simulink model "PV_Boost_VSI_Ilhamento_SMS_2023b"  (R2024b)
settings: Solver=ode4  StartTime=0  StopTime=5  FixedStep=1e-6  MaxStep=1e-6  RelTol=0.1e-3
undefined symbols (not defined in the file): Cl, Ll, Rl
libraries: spsSeriesRLCBranchLib x7, spsIGBTDiodeLib x5, spsGroundLib x4, spsVoltageMeasurementLib x4, slpidlib x3, simulink x3, spsBreakerLib x2, spsCurrentMeasurementLib x2, spsDiodeLib x2, spsMeanLib x2, spsACVoltageSourceLib x1, spsParallelRLCBranchLib x1
settings Model: SimulationMode=accelerator  Creator=rodrigo  LastModifiedBy=aleks
settings SolverCC: MaxConsecutiveZCs=10000  ShapePreserveControl=EnableAll  ZeroCrossControl=EnableAll
settings DataIOCC: SaveFormat=Array  SignalLoggingSaveFormat=ModelDataLogs  SaveOutput=off  SaveTime=off  ReturnWorkspaceOutputs=off
settings OptimizationCC: BooleanDataType=off  ExpressionDepthLimit=2147483647  InitFltsAndDblsToZero=on  EfficientMapNaN2IntZero=off  LifeSpan=inf  AccelVerboseBuild=on
settings DebuggingCC: SaveWithParameterizedLinksMsg=none  UnderspecifiedInitializationDetection=Classic  MergeDetectMultiDrivingBlocksExec=none  SignalResolutionControl=TryResolveAllWithWarning  MultiTaskDSMMsg=warning  MultiTaskCondExecSysMsg=none  FcnCallInpInsideContextMsg=warning  UnconnectedInputMsg=warning  UnconnectedOutputMsg=warning  UnconnectedLineMsg=warning  StateNameClashWarn=warning  StrictBusMsg=WarnOnBusTreatedAsVector  SFUnexpectedBacktrackingDiag=warning  SFNoUnconditionalDefaultTransitionDiag=warning  SFExecutionAtInitializationDiag=none  ArithmeticOperatorsInVariantConditions=warning
settings HardwareCC: ProdBitPerPointer=32  ProdBitPerSizeT=32  ProdBitPerPtrDiffT=32  ProdLargestAtomicFloat=None  ProdIntDivRoundTo=Undefined  ProdEndianess=Unspecified  ProdWordSize=32  ProdHWDeviceType=32-bit Generic  TargetBitPerPointer=64  TargetBitPerSizeT=64  TargetBitPerPtrDiffT=64  TargetLongLongMode=on  TargetIntDivRoundTo=Zero  TargetEndianess=LittleEndian  TargetWordSize=64  TargetHWDeviceType=MATLAB Host  ProdEqTarget=off
settings ModelReferenceCC: PropagateSignalLabelsOutOfModel=off
settings SFSimCC: SimUseLocalCustomCode=off  SimParseCustomCode=off  CustomCodeUndefinedFunction=UseInterfaceOnly
settings RTWCC: RTWUseLocalCustomCode=off  GPUComputeCapability=3.5
settings CodeAppCC: MaxIdLength=128  StateflowObjectComments=on
settings GRTTargetCC: TargetLangStandard=C89/C90 (ANSI)  CombineOutputUpdateFcns=off  GRTInterface=on
settings ConfigComp: CovMetricSettings=dw  CovSaveCumulativeToWorkspaceVar=on  CovSaveSingleToWorkspaceVar=on  CovExternalEMLEnable=off  DVMaxTestCaseSteps=500  DVTestSuiteOptimization=CombinedObjectives (Nonlinear Extended)  DVDefectChecker=off  DVDetectActiveLogic=on  DVHarnessSource=Signal Editor
settings SimscapeCC: SimscapeNormalizeSystem=off

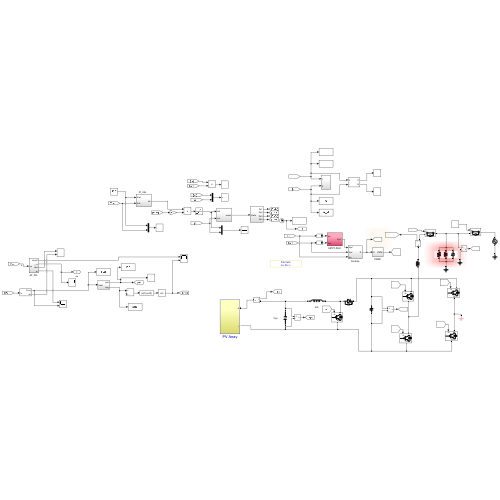
[thumbnail: Simulink's stored preview of the top-level diagram]
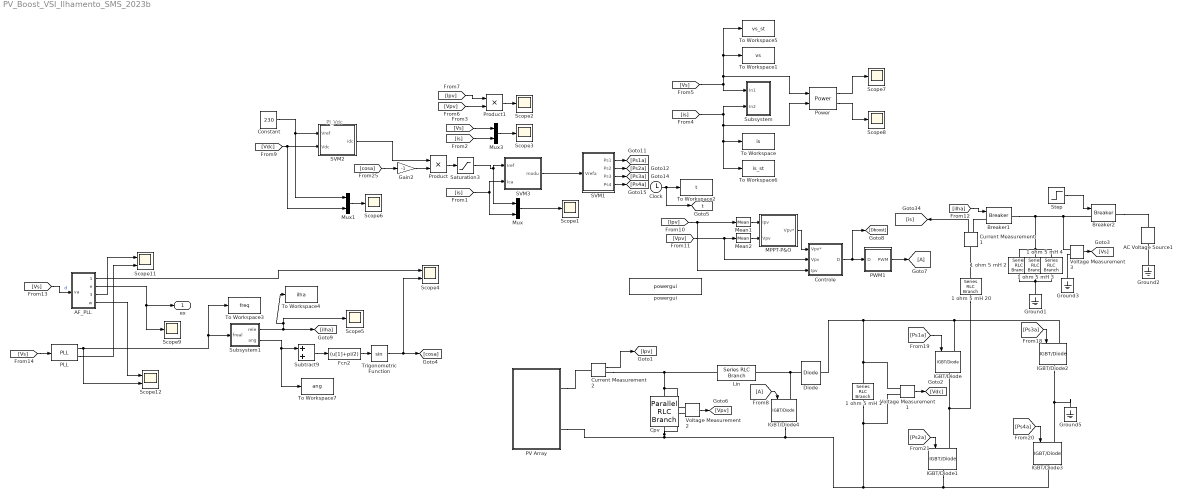
== system PV_Boost_VSI_Ilhamento_SMS_2023b ==
  note: PI_Vdc
  1 ohm 5 mH 1 : spsSeriesRLCBranchLib/Series RLC Branch  LConnTagsString=__new0  RConnTagsString=__new0  BranchType=C  Resistance=100  Inductance=0.547e-3  SetiL0=off  InitialCurrent=10  Capacitance=0.002115  Setx0=on  InitialVoltage=230  Measurements=None
  1 ohm 5 mH 2 : spsSeriesRLCBranchLib/Series RLC Branch  LConnTagsString=__new0  RConnTagsString=__new0  BranchType=R  Resistance=Rl  Inductance=5e-03  SetiL0=off  InitialCurrent=0  Capacitance=0.001  Setx0=off  InitialVoltage=0  Measurements=None
  1 ohm 5 mH 20 : spsSeriesRLCBranchLib/Series RLC Branch  LConnTagsString=__new0  RConnTagsString=__new0  BranchType=L  Resistance=100  Inductance=1.5e-3  SetiL0=off  InitialCurrent=10  Capacitance=60u  Setx0=off  InitialVoltage=0  Measurements=None
  1 ohm 5 mH 3 : spsSeriesRLCBranchLib/Series RLC Branch  LConnTagsString=__new0  RConnTagsString=__new0  BranchType=L  Resistance=100  Inductance=Ll  SetiL0=off  InitialCurrent=10  Capacitance=60u  Setx0=off  InitialVoltage=0  Measurements=None
  1 ohm 5 mH 4 : spsSeriesRLCBranchLib/Series RLC Branch  LConnTagsString=__new0  RConnTagsString=__new0  BranchType=C  Resistance=100  Inductance=0.547e-3  SetiL0=off  InitialCurrent=10  Capacitance=Cl  Setx0=off  InitialVoltage=230  Measurements=None
  AC Voltage Source1 : spsACVoltageSourceLib/AC Voltage Source  Amplitude=127*sqrt(2)  Phase=0  Frequency=60  SampleTime=0  Measurements=None  BusType=swing  Pref=10e3  Qref=0  Qmin=-inf  Qmax=+inf
  AF_PLL : Subsystem
  Breaker1 : spsBreakerLib/Breaker  InitialState=1  SwitchingTimes="[1/60  5/60]"  External=on  BreakerResistance=0.0001  SnubberResistance=1e6  SnubberCapacitance=inf  Measurements=None  MoreParameters=on  NoBreakLoop=off
  Breaker2 : spsBreakerLib/Breaker  InitialState=1  SwitchingTimes="[1/60  5/60]"  External=on  BreakerResistance=0.0001  SnubberResistance=1e6  SnubberCapacitance=inf  Measurements=None  MoreParameters=on  NoBreakLoop=off
  Clock : Clock
  Constant : Constant  Value=230  SampleTime=-1
  Controle : Subsystem
  Cpv : spsParallelRLCBranchLib/Parallel RLC Branch  LConnTagsString=a  RConnTagsString=__new0  BranchType=C  Resistance=1  Inductance=1e-3  SetiL0=off  InitialCurrent=0  Capacitance=100e-6  Setx0=off  InitialVoltage=0  Measurements=Branch voltage
  Current Measurement1 : spsCurrentMeasurementLib/Current Measurement  PhasorSimulation=off  OutputType=Complex  PSBequivalent=0
  Current Measurement2 : spsCurrentMeasurementLib/Current Measurement  PhasorSimulation=off  OutputType=Complex  PSBequivalent=0
  Diode : spsDiodeLib/Diode  Ron=0.001  Lon=0  Vf=0.0  IC=0  UseSnubber=off  Rs=500  Cs=250e-9  Measurements=off
  Fcn2 : Fcn  Expr=(u[1]+pi/2)
  From8 : From
  Gain2 : Gain  Gain=-1
  Goto7 : Goto
  Ground{1..3,5} (4 alike) : spsGroundLib/Ground  LConnTagsString=a
  IGBT/Diode{,1..4} (5 alike) : spsIGBTDiodeLib/IGBT//Diode  Ron=1e-3  Rs=1e5  Cs=inf  Measurements=off
  Lin : spsSeriesRLCBranchLib/Series RLC Branch  LConnTagsString=__new0  RConnTagsString=__new0  BranchType=L  Resistance=0.01  Inductance=2.5e-3  SetiL0=off  InitialCurrent=0  Capacitance=1e-6  Setx0=off  InitialVoltage=0  Measurements=Branch current
  MPPT-P&O : Subsystem
  Mean1 : spsMeanLib/Mean  Freq=200  Vinit=0  Ts=0
  Mean2 : spsMeanLib/Mean  Freq=200  Vinit=0  Ts=0
  Mux : Mux  Inputs=2
  Mux1 : Mux  Inputs=2
  Mux3 : Mux  Inputs=2
  PLL : spsPLLLib/PLL  Fmin=45  Par_Init=[0, 60]  ParK=[180, 3200, 1]  TcD=1e-4  MaxRateChangeFreq=12  FilterCutOffFreq=25  Ts=0  AGC=on
      settings: LibrarySourceBlock=sps_lib/Control/PLL
  PV Array : Subsystem
  PWM1 : Subsystem
  Power : spsPowerLib/Power  Freq=60  Vinit=[1, 0]  Iinit=[1, 0]  Ts=0
  Product : Product  RndMeth=Zero
  Product1 : Product  RndMeth=Zero
  SVM1 : Subsystem
  SVM2 : Subsystem
  SVM3 : Subsystem
  Saturation3 : Saturate  UpperLimit=1000  LowerLimit=-100  LinearizeAsGain=off
  Scope{1..3,5..9} (8 alike) : Scope
  Scope11 : Scope  NumInputPorts=2
  Scope12 : Scope  NumInputPorts=2
  Scope4 : Scope  NumInputPorts=2
  Step : Step  Time=3  Before=1  After=0  SampleTime=0
  Subsystem : Subsystem
  Subsystem1 : Subsystem
  Subtract9 : Sum
  To Workspace : ToWorkspace  VariableName=is  SampleTime=-1
      settings: Decimation=100
  To Workspace1 : ToWorkspace  VariableName=vs  SampleTime=-1
      settings: Decimation=100
  To Workspace2 : ToWorkspace  VariableName=t  SampleTime=1e-6
      settings: Decimation=100
  To Workspace3 : ToWorkspace  VariableName=freq  SampleTime=-1
      settings: Decimation=100
  To Workspace4 : ToWorkspace  VariableName=ilha  SampleTime=-1
      settings: Decimation=100
  To Workspace5 : ToWorkspace  VariableName=vs_st  SaveFormat=Structure With Time  SampleTime=-1
      settings: Decimation=100
  To Workspace6 : ToWorkspace  VariableName=is_st  SaveFormat=Structure With Time  SampleTime=-1
      settings: Decimation=100
  To Workspace7 : ToWorkspace  VariableName=ang  SampleTime=-1
      settings: Decimation=100
  Trigonometric Function : Trigonometry
  Voltage Measurement1 : spsVoltageMeasurementLib/Voltage Measurement  PhasorSimulation=off  OutputType=Complex  PSBequivalent=0
  Voltage Measurement2 : spsVoltageMeasurementLib/Voltage Measurement  PhasorSimulation=off  OutputType=Complex  PSBequivalent=0
  Voltage Measurement3 : spsVoltageMeasurementLib/Voltage Measurement  PhasorSimulation=off  OutputType=Complex  PSBequivalent=0
  powergui : spspowerguiLib/powergui  Priority=1  SimulationMode=Discrete  SampleTime=1e-6  frequency=60  Iterations=50  frequencyindice=0  Pbase=100e6  ErrMax=1e-4  UnitsV=kV  UnitsW=MW  buscounter=0  FunctionMessages=off  echomessages=off  EnableUseOfTLC=off  CurrentSourceSwitches=off  DisableSnubberDevices=off  DisableRonSwitches=off  DisableVfSwitches=off  DisplayEquations=off  AutomaticDiscreteSolvers=off  SolverType=Tustin  Interpol=off  ExternalGateDelay=off  methode=off  Ts=0  x0status=blocks  SPID=on  SwTol=0  HookPort=off  NonlinearTolerance=1e-4  nMaxIteration=100  ContinueOnMaxIteration=off  RestoreLinks=warning  ResistiveCurrentMeasurement=off  Frange=[0:2:500]  Ylog=off  Xlog=on  ShowGrid=off  save=off  variable=ZData  structure=fft  ZoomFFT=on  StartTime=1  cycles=5  DisplayStyle=2  fundamental=60  FreqAxis=on  MaxFrequency=51*60  frequencyindicesteady=1  RmsSteady=1  display=off
  ex : Outport
  tag scope: t=global
  wires:
  [Ps3a] -> IGBT/Diode2/1
  [Ps1a] -> IGBT/Diode/1
  [Ps4a] -> IGBT/Diode3/1
  [Ps2a] -> IGBT/Diode1/1
  SVM1/1(Ps1) -> [Ps1a]
  SVM1/2(Ps2) -> [Ps2a]
  SVM1/3(Ps3) -> [Ps3a]
  SVM1/4(Ps4) -> [Ps4a]
  Voltage Measurement1/1 -> [Vdc]
  [Vdc] -> Mux1/2, SVM2/2(Vdc)
  Saturation3/1 -> SVM3/1(Iref), Mux/1
  Mux/1 -> Scope1/1
  [is] -> Mux/2, SVM3/2(Ica)
  Mux1/1 -> Scope6/1
  Constant/1 -> Mux1/1, SVM2/1(Vref)
  Current Measurement1/1 -> [is]
  Mux3/1 -> Scope3/1
  [is] -> Mux3/2
  Current Measurement2/1 -> [Ipv]
  [Vs] -> Mux3/1
  Product1/1 -> Scope2/1
  [Vpv] -> Product1/2
  [Ipv] -> Product1/1
  From8/1 -> IGBT/Diode4/1
  Voltage Measurement2/1 -> [Vpv]
  Product/1 -> Saturation3/1
  SVM2/1(idc) -> Product/1
  [Vpv] -> Controle/2(Vpv), Mean2/1
  [Ipv] -> Controle/3(Ipv), Mean1/1
  Controle/1(D) -> [Dboost], PWM1/1(D)
  MPPT-P&O/1(Vpv*) -> Controle/1(Vpv*)
  Mean2/1 -> MPPT-P&O/2(Vpv)
  Mean1/1 -> MPPT-P&O/1(Ipv)
  PWM1/1(PWM) -> Goto7/1
  Step/1 -> Breaker2/1
  [Vs] -> To Workspace5/1, To Workspace1/1, Power/1, Subsystem/1(In1)
  [is] -> Subsystem/2(In2), Power/2, To Workspace/1, To Workspace6/1
  Clock/1 -> [t], To Workspace2/1
  [Vs] -> PLL/1
  Gain2/1 -> Product/2
  SVM3/1(modu) -> SVM1/1(Vrefa)
  Trigonometric Function/1 -> [cosa], Scope4/2
  [cosa] -> Gain2/1
  Subsystem1/1(rele) -> To Workspace4/1, Scope5/1, [ilha]
  Power/1 -> Scope7/1
  Power/2 -> Scope8/1
  Subsystem1/2(ang) -> Subtract9/1, To Workspace7/1
  [Vs] -> AF_PLL/1(va)  "d"
  AF_PLL/1(cosa2) -> Scope4/1
  AF_PLL/2(e) -> Scope9/1, ex/1
  Voltage Measurement3/1 -> [Vs]
  [ilha] -> Breaker1/1
  PLL/2 -> Scope11/2
  AF_PLL/4(w) -> Scope12/1
  Subtract9/1 -> Fcn2/1
  Fcn2/1 -> Trigonometric Function/1
  PLL/1 -> To Workspace3/1, Subsystem1/1(freal), Scope12/2
  AF_PLL/3(teta) -> Scope11/1
  connections:
  IGBT/Diode2/RConn1 -- Ground5/LConn1 -- IGBT/Diode3/LConn1
  IGBT/Diode1/LConn1 -- 1 ohm 5 mH 20/LConn1 -- IGBT/Diode/RConn1
  1 ohm 5 mH 20/RConn1 -- Current Measurement1/LConn1
  1 ohm 5 mH 1/LConn1 -- Diode/RConn1 -- IGBT/Diode2/LConn1 -- IGBT/Diode/LConn1 -- Voltage Measurement1/LConn1
  IGBT/Diode1/RConn1 -- IGBT/Diode3/RConn1 -- Voltage Measurement1/LConn2 -- 1 ohm 5 mH 1/RConn1 -- IGBT/Diode4/RConn1 -- Voltage Measurement2/LConn2 -- Cpv/RConn1 -- PV Array/RConn2
  Ground2/LConn1 -- AC Voltage Source1/LConn1
  Diode/LConn1 -- IGBT/Diode4/LConn1 -- Lin/RConn1
  Lin/LConn1 -- Current Measurement2/RConn1 -- Voltage Measurement2/LConn1 -- Cpv/LConn1
  PV Array/RConn1 -- Current Measurement2/LConn1
  1 ohm 5 mH 2/LConn1 -- 1 ohm 5 mH 4/RConn1 -- 1 ohm 5 mH 3/RConn1 -- Ground1/LConn1
  Ground3/LConn1 -- Voltage Measurement3/LConn2
  Breaker2/RConn1 -- AC Voltage Source1/RConn1
  Breaker1/LConn1 -- Current Measurement1/RConn1
  1 ohm 5 mH 4/LConn1 -- Breaker1/RConn1 -- Breaker2/LConn1 -- Voltage Measurement3/LConn1 -- 1 ohm 5 mH 2/RConn1 -- 1 ohm 5 mH 3/LConn1

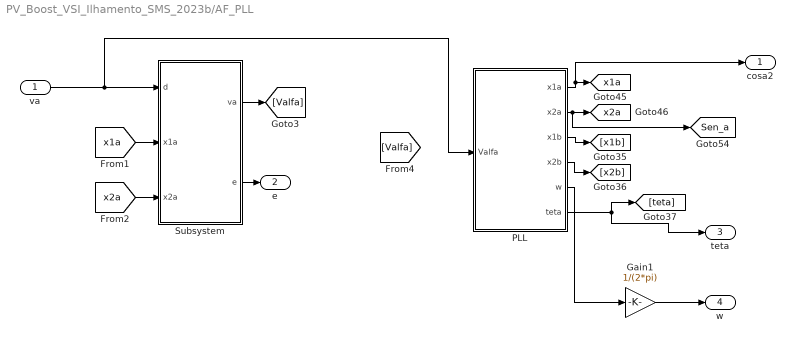
== system PV_Boost_VSI_Ilhamento_SMS_2023b/AF_PLL ==
  va : Inport
  Gain1 : Gain  Gain=1/(2*pi)
  PLL : Subsystem
  Subsystem : Subsystem
  cosa2 : Outport
  e : Outport  Port=2
  teta : Outport  Port=3
  w : Outport  Port=4
  tag scope: Sen_a=global, x1a=global, x2a=global
  wires:
  Subsystem/1(va) -> [Valfa]
  PLL/1(x1a) -> cosa2/1, [x1a]
  va/1 -> PLL/1(Valfa), Subsystem/1(d)
  PLL/6(teta) -> [teta], teta/1
  [x2a] -> Subsystem/3(x2a)
  PLL/3(x1b) -> [x1b]
  PLL/4(x2b) -> [x2b]
  [x1a] -> Subsystem/2(x1a)
  Subsystem/2(e) -> e/1
  PLL/2(x2a) -> [Sen_a], [x2a]
  PLL/5(w) -> Gain1/1
  Gain1/1 -> w/1

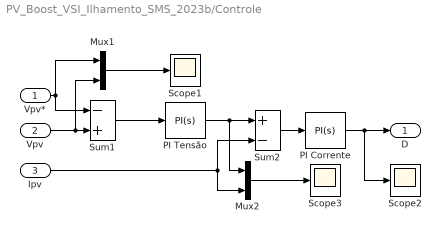
== system PV_Boost_VSI_Ilhamento_SMS_2023b/Controle ==
  Vpv* : Inport
  Vpv : Inport  Port=2
  Ipv : Inport  Port=3
  Mux1 : Mux  Inputs=2
  Mux2 : Mux  Inputs=2
  PI Corrente : slpidlib/PID Controller  Controller=PI  Form=Parallel  TimeDomain=Continuous-time  UseExternalTs=off  SampleTime=-1  IntegratorMethod=Forward Euler  FilterMethod=Forward Euler  ControllerParametersSource=internal  P=0.0057  I=19.4970  UseKiTs=off  D=0  UseExternalDerivativeSource=off  N=100  UseFilter=on  TunerSelectOption=Transfer Function Based (PID Tuner App)  InitialConditionSource=internal  InitialConditionForIntegrator=0  InitialConditionForFilter=0  DifferentiatorICPrevScaledInput=0  ExternalReset=none  TrackingMode=off  Kt=1  LimitOutput=on  SatLimitsSource=internal  UpperSaturationLimit=0.95  LowerSaturationLimit=0  LinearizeAsGain=on  AntiWindupMode=none  Kb=1  LimitIntegrator=off  UpperIntegratorSaturationLimit=inf  LowerIntegratorSaturationLimit=-inf  POutMin=[]  POutMax=[]  IOutMin=[]  IOutMax=[]  DOutMin=[]  DOutMax=[]  NOutMin=[]  NOutMax=[]  SumOutMin=[]  SumOutMax=[]  SaturationOutMin=[]  SaturationOutMax=[]  PParamMin=[]  PParamMax=[]  IParamMin=[]  IParamMax=[]  DParamMin=[]  DParamMax=[]  NParamMin=[]  NParamMax=[]  KbParamMin=[]  KbParamMax=[]  KtParamMin=[]  KtParamMax=[]  KbOutMin=[]  KbOutMax=[]  KtOutMin=[]  KtOutMax=[]  IntegratorOutMin=[]  IntegratorOutMax=[]  FilterOutMin=[]  FilterOutMax=[]  SumI1OutMin=[]  SumI1OutMax=[]  SumI2OutMin=[]  SumI2OutMax=[]  SumI3OutMin=[]  SumI3OutMax=[]  SumI4OutMin=[]  SumI4OutMax=[]  SumDOutMin=[]  SumDOutMax=[]  DifferentiatorOutMin=[]  DifferentiatorOutMax=[]  FilterDiffOutCoefMin=[]  FilterDiffOutCoefMax=[]  ReciprocalOutMin=[]  ReciprocalOutMax=[]  SumDenOutMin=[]  SumDenOutMax=[]  SumNumOutMin=[]  SumNumOutMax=[]  DivideOutMin=[]  DivideOutMax=[]  UdiffTsProdOutMin=[]  UdiffTsProdOutMax=[]  NTsProdOutMin=[]  NTsProdOutMax=[]  UintegralTsProdOutMin=[]  UintegralTsProdOutMax=[]  UngainTsProdOutMin=[]  UngainTsProdOutMax=[]  ClampingZeroOutDataTypeStr=Inherit: Inherit via back propagation  ClampingZeroOutMin=[]  ClampingZeroOutMax=[]  FilterDenConstantOutDataTypeStr=Inherit: Inherit via back propagation  FilterDenConstantOutMin=[]  FilterDenConstantOutMax=[]  PCopyOutDataTypeStr=Inherit: Inherit via back propagation  PCopyOutMin=[]  PCopyOutMax=[]  NCopyOutDataTypeStr=Inherit: Inherit via back propagation  NCopyOutMin=[]  NCopyOutMax=[]  IntegratorContinuousStateAttributes=''  IntegratorStateMustResolveToSignalObject=off  IntegratorRTWStateStorageClass=Auto  FilterContinuousStateAttributes=''  FilterStateMustResolveToSignalObject=off  FilterRTWStateStorageClass=Auto  ParallelPVariant=InternalParameters  IdealPVariant=Disabled  IVariant=InternalParameters  DVariant=Disabled  IntegratorVariant=Continuous  SatVariant=Enabled  AWVariant=Passthrough  PCopyVariant=Disabled  TRVariant=Disabled  FdbkBlocksVariant=Forward  IdealPFdbkVariant=Disabled  SatFdbkVariant=Disabled  DerivativeFilterVariant=Disabled  NVariant=Disabled  NCopyVariant=Disabled_SignalSpec  FilterICVariant=Disabled  IntegratorICVariant=InternalICs  ExternalResetVariant=Disabled  TRSumVariant=Passthrough  SumFdbkVariant=Disabled  SumVariant=Sum_PI  TsampFilterVariant=InternalTs  TsampNgainVariant=Passthrough  TsampIntegralVariant=Disabled_SignalSpec  ExternalSaturationOutDataTypeStr=Inherit: Same as second input  DerivativeSourceVariant=Disabled  PreIntVariant=InternalPreInt
  PI Tensão : slpidlib/PID Controller  Controller=PI  Form=Parallel  TimeDomain=Continuous-time  UseExternalTs=off  SampleTime=-1  IntegratorMethod=Forward Euler  FilterMethod=Forward Euler  ControllerParametersSource=internal  P=0.0351  I=24.45  UseKiTs=off  D=0  UseExternalDerivativeSource=off  N=100  UseFilter=on  TunerSelectOption=Transfer Function Based (PID Tuner App)  InitialConditionSource=internal  InitialConditionForIntegrator=0  InitialConditionForFilter=0  DifferentiatorICPrevScaledInput=0  ExternalReset=none  TrackingMode=off  Kt=1  LimitOutput=on  SatLimitsSource=internal  UpperSaturationLimit=10  LowerSaturationLimit=0  LinearizeAsGain=on  AntiWindupMode=none  Kb=1  LimitIntegrator=off  UpperIntegratorSaturationLimit=inf  LowerIntegratorSaturationLimit=-inf  POutMin=[]  POutMax=[]  IOutMin=[]  IOutMax=[]  DOutMin=[]  DOutMax=[]  NOutMin=[]  NOutMax=[]  SumOutMin=[]  SumOutMax=[]  SaturationOutMin=[]  SaturationOutMax=[]  PParamMin=[]  PParamMax=[]  IParamMin=[]  IParamMax=[]  DParamMin=[]  DParamMax=[]  NParamMin=[]  NParamMax=[]  KbParamMin=[]  KbParamMax=[]  KtParamMin=[]  KtParamMax=[]  KbOutMin=[]  KbOutMax=[]  KtOutMin=[]  KtOutMax=[]  IntegratorOutMin=[]  IntegratorOutMax=[]  FilterOutMin=[]  FilterOutMax=[]  SumI1OutMin=[]  SumI1OutMax=[]  SumI2OutMin=[]  SumI2OutMax=[]  SumI3OutMin=[]  SumI3OutMax=[]  SumI4OutMin=[]  SumI4OutMax=[]  SumDOutMin=[]  SumDOutMax=[]  DifferentiatorOutMin=[]  DifferentiatorOutMax=[]  FilterDiffOutCoefMin=[]  FilterDiffOutCoefMax=[]  ReciprocalOutMin=[]  ReciprocalOutMax=[]  SumDenOutMin=[]  SumDenOutMax=[]  SumNumOutMin=[]  SumNumOutMax=[]  DivideOutMin=[]  DivideOutMax=[]  UdiffTsProdOutMin=[]  UdiffTsProdOutMax=[]  NTsProdOutMin=[]  NTsProdOutMax=[]  UintegralTsProdOutMin=[]  UintegralTsProdOutMax=[]  UngainTsProdOutMin=[]  UngainTsProdOutMax=[]  ClampingZeroOutDataTypeStr=Inherit: Inherit via back propagation  ClampingZeroOutMin=[]  ClampingZeroOutMax=[]  FilterDenConstantOutDataTypeStr=Inherit: Inherit via back propagation  FilterDenConstantOutMin=[]  FilterDenConstantOutMax=[]  PCopyOutDataTypeStr=Inherit: Inherit via back propagation  PCopyOutMin=[]  PCopyOutMax=[]  NCopyOutDataTypeStr=Inherit: Inherit via back propagation  NCopyOutMin=[]  NCopyOutMax=[]  IntegratorContinuousStateAttributes=''  IntegratorStateMustResolveToSignalObject=off  IntegratorRTWStateStorageClass=Auto  FilterContinuousStateAttributes=''  FilterStateMustResolveToSignalObject=off  FilterRTWStateStorageClass=Auto  ParallelPVariant=InternalParameters  IdealPVariant=Disabled  IVariant=InternalParameters  DVariant=Disabled  IntegratorVariant=Continuous  SatVariant=Enabled  AWVariant=Passthrough  PCopyVariant=Disabled  TRVariant=Disabled  FdbkBlocksVariant=Forward  IdealPFdbkVariant=Disabled  SatFdbkVariant=Disabled  DerivativeFilterVariant=Disabled  NVariant=Disabled  NCopyVariant=Disabled_SignalSpec  FilterICVariant=Disabled  IntegratorICVariant=InternalICs  ExternalResetVariant=Disabled  TRSumVariant=Passthrough  SumFdbkVariant=Disabled  SumVariant=Sum_PI  TsampFilterVariant=InternalTs  TsampNgainVariant=Passthrough  TsampIntegralVariant=Disabled_SignalSpec  ExternalSaturationOutDataTypeStr=Inherit: Same as second input  DerivativeSourceVariant=Disabled  PreIntVariant=InternalPreInt
  Scope1 : Scope
  Scope2 : Scope
  Scope3 : Scope
  Sum1 : Sum  Inputs=-+  InputSameDT=on  SaturateOnIntegerOverflow=on  OutDataTypeStr=Inherit: Same as first input
  Sum2 : Sum  Inputs=+-  InputSameDT=on  SaturateOnIntegerOverflow=on  OutDataTypeStr=Inherit: Same as first input
  D : Outport
  wires:
  Mux1/1 -> Scope1/1
  Mux2/1 -> Scope3/1
  Ipv/1 -> Sum2/2, Mux2/2
  Sum2/1 -> PI Corrente/1
  PI Corrente/1 -> Scope2/1, D/1
  PI Tensão/1 -> Mux2/1, Sum2/1
  Vpv*/1 -> Mux1/1, Sum1/1
  Sum1/1 -> PI Tensão/1
  Vpv/1 -> Mux1/2, Sum1/2

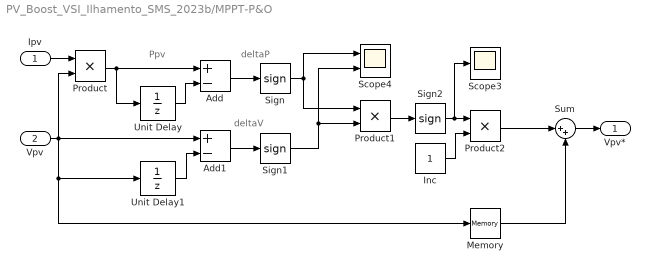
== system PV_Boost_VSI_Ilhamento_SMS_2023b/MPPT-P&O ==
  note: deltaV
  note: deltaP
  note: Ppv
  Ipv : Inport
  Vpv : Inport  Port=2
  Add : Sum  Inputs=+-
  Add1 : Sum  Inputs=+-
  Inc : Constant
  Memory : Memory  InheritSampleTime=on
  Product : Product
  Product1 : Product
  Product2 : Product
  Scope3 : Scope
  Scope4 : Scope  NumInputPorts=2
  Sign : Signum
  Sign1 : Signum
  Sign2 : Signum
  Sum : Sum  Inputs=|++
  Unit Delay : UnitDelay  SampleTime=-1  HasFrameUpgradeWarning=on
  Unit Delay1 : UnitDelay  SampleTime=-1  HasFrameUpgradeWarning=on
  Vpv* : Outport
  wires:
  Add/1 -> Sign/1
  Add1/1 -> Sign1/1
  Product1/1 -> Sign2/1
  Sign2/1 -> Scope3/1, Product2/1
  Inc/1 -> Product2/2
  Product2/1 -> Sum/1
  Sum/1 -> Vpv*/1
  Unit Delay/1 -> Add/2
  Unit Delay1/1 -> Add1/2
  Product/1 -> Unit Delay/1, Add/1
  Ipv/1 -> Product/1
  Memory/1 -> Sum/2
  Vpv/1 -> Memory/1, Unit Delay1/1, Product/2, Add1/1
  Sign/1 -> Scope4/1, Product1/1
  Sign1/1 -> Scope4/2, Product1/2

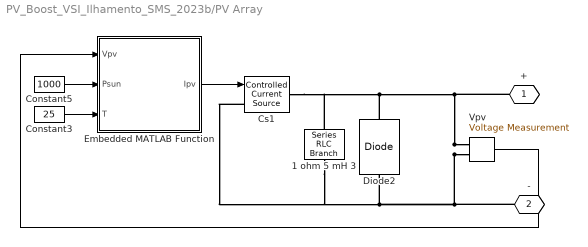
== system PV_Boost_VSI_Ilhamento_SMS_2023b/PV Array ==
  1 ohm 5 mH 3 : spsSeriesRLCBranchLib/Series RLC Branch  LConnTagsString=__new0  RConnTagsString=__new0  BranchType=C  Resistance=100  Inductance=0.547e-3  SetiL0=off  InitialCurrent=10  Capacitance=100e-6  Setx0=off  InitialVoltage=123.2  Measurements=Branch voltage
  Constant3 : Constant  Value=25
  Constant5 : Constant  Value=1000
  Cs1 : spsControlledCurrentSourceLib/Controlled Current Source  Initialize=on  Source_Type=DC  Amplitude=0  Phase=0  Frequency=0  Measurements=None
  Diode2 : spsDiodeLib/Diode  Ron=0.001  Lon=0  Vf=0  IC=0  UseSnubber=off  Rs=10000000000000  Cs=250e-9  Measurements=off
  Embedded MATLAB Function : MATLAB Function  TreatAsAtomicUnit=on
  Vpv : spsVoltageMeasurementLib/Voltage Measurement  PhasorSimulation=off  OutputType=Complex  PSBequivalent=0
  + : PMIOPort  Tag=PMCPort  Side=Right
  - : PMIOPort  Tag=PMCPort  Port=2  Side=Right
  wires:
  Vpv/1 -> Embedded MATLAB Function/1(Vpv)
  Constant3/1 -> Embedded MATLAB Function/3(T)
  Constant5/1 -> Embedded MATLAB Function/2(Psun)
  Embedded MATLAB Function/1(Ipv) -> Cs1/1
  connections:
  Vpv/LConn1 -- +/RConn1 -- Cs1/RConn1 -- 1 ohm 5 mH 3/LConn1 -- Diode2/RConn1
  Vpv/LConn2 -- -/RConn1 -- Cs1/LConn1 -- 1 ohm 5 mH 3/RConn1 -- Diode2/LConn1

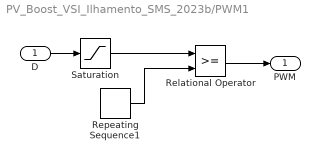
== system PV_Boost_VSI_Ilhamento_SMS_2023b/PWM1 ==
  D : Inport
  Relational Operator : RelationalOperator  OutDataTypeStr=boolean  InputSameDT=off
  Repeating Sequence1 : simulink/Sources/Repeating Sequence  rep_seq_t=[0 1]/20e3  rep_seq_y=[0 1]
  Saturation : Saturate  UpperLimit=1  LowerLimit=0
  PWM : Outport
  wires:
  D/1 -> Saturation/1
  Repeating Sequence1/1 -> Relational Operator/2
  Relational Operator/1 -> PWM/1
  Saturation/1 -> Relational Operator/1

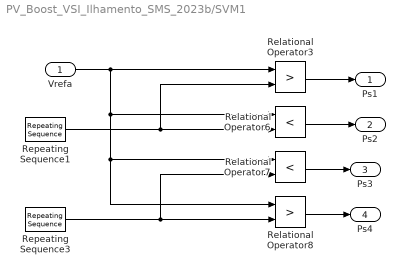
== system PV_Boost_VSI_Ilhamento_SMS_2023b/SVM1 ==
  Vrefa : Inport
  Relational Operator3 : RelationalOperator  Operator=>  OutDataTypeStr=boolean  InputSameDT=off
  Relational Operator6 : RelationalOperator  Operator=<  OutDataTypeStr=boolean  InputSameDT=off
  Relational Operator7 : RelationalOperator  Operator=<  OutDataTypeStr=boolean  InputSameDT=off
  Relational Operator8 : RelationalOperator  Operator=>  OutDataTypeStr=boolean  InputSameDT=off
  Repeating Sequence1 : simulink/Sources/Repeating Sequence  rep_seq_t=[0 1/(2*20e3) 1/20e3]  rep_seq_y=[0 1 0]
  Repeating Sequence3 : simulink/Sources/Repeating Sequence  rep_seq_t=[0 1/(2*20e3) 1/20e3]  rep_seq_y=[1 0 1]
  Ps1 : Outport
  Ps2 : Outport  Port=2
  Ps3 : Outport  Port=3
  Ps4 : Outport  Port=4
  wires:
  Vrefa/1 -> Relational Operator3/1, Relational Operator7/1, Relational Operator8/1, Relational Operator6/1
  Repeating Sequence1/1 -> Relational Operator6/2, Relational Operator3/2
  Repeating Sequence3/1 -> Relational Operator8/2, Relational Operator7/2
  Relational Operator3/1 -> Ps1/1
  Relational Operator6/1 -> Ps2/1
  Relational Operator7/1 -> Ps3/1
  Relational Operator8/1 -> Ps4/1

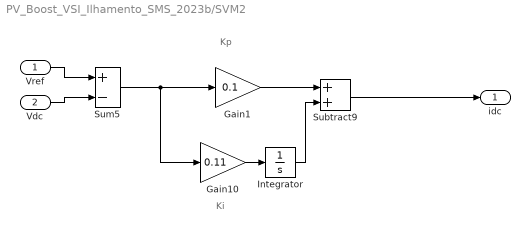
== system PV_Boost_VSI_Ilhamento_SMS_2023b/SVM2 ==
  note: Ki
  note: Kp
  Vref : Inport
  Vdc : Inport  Port=2
  Gain1 : Gain  Gain=0.1
  Gain10 : Gain  Gain=0.11
  Integrator : Integrator
  Subtract9 : Sum
  Sum5 : Sum  Inputs=+-  InputSameDT=on  SaturateOnIntegerOverflow=on  OutDataTypeStr=Inherit: Same as first input
  idc : Outport
  wires:
  Vdc/1 -> Sum5/2
  Gain1/1 -> Subtract9/1
  Gain10/1 -> Integrator/1
  Integrator/1 -> Subtract9/2
  Sum5/1 -> Gain1/1, Gain10/1
  Vref/1 -> Sum5/1
  Subtract9/1 -> idc/1

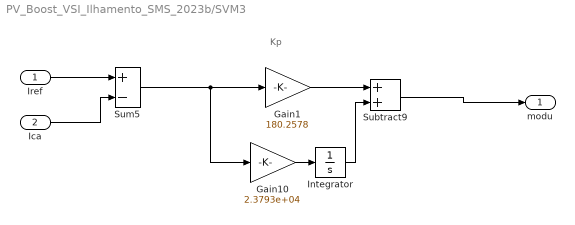
== system PV_Boost_VSI_Ilhamento_SMS_2023b/SVM3 ==
  note: Kp
  Iref : Inport
  Ica : Inport  Port=2
  Gain1 : Gain  Gain=180.2578
  Gain10 : Gain  Gain=2.3793e+04
  Integrator : Integrator
  Subtract9 : Sum
  Sum5 : Sum  Inputs=+-  InputSameDT=on  SaturateOnIntegerOverflow=on  OutDataTypeStr=Inherit: Same as first input
  modu : Outport
  wires:
  Iref/1 -> Sum5/1
  Ica/1 -> Sum5/2
  Gain1/1 -> Subtract9/1
  Gain10/1 -> Integrator/1
  Integrator/1 -> Subtract9/2
  Sum5/1 -> Gain1/1, Gain10/1
  Subtract9/1 -> modu/1

== system PV_Boost_VSI_Ilhamento_SMS_2023b/Subsystem ==
  In1 : Inport
  In2 : Inport  Port=2
  RMS : spsRMSLib/RMS  TrueRMS=on  Freq=60  RMSInit=127  Ts=0
  Scope1 : Scope
  To Workspace1 : ToWorkspace  VariableName=vsef  SampleTime=-1
      settings: Decimation=100
  wires:
  In2/1 -> ?
  RMS/1 -> To Workspace1/1, Scope1/1
  In1/1 -> RMS/1

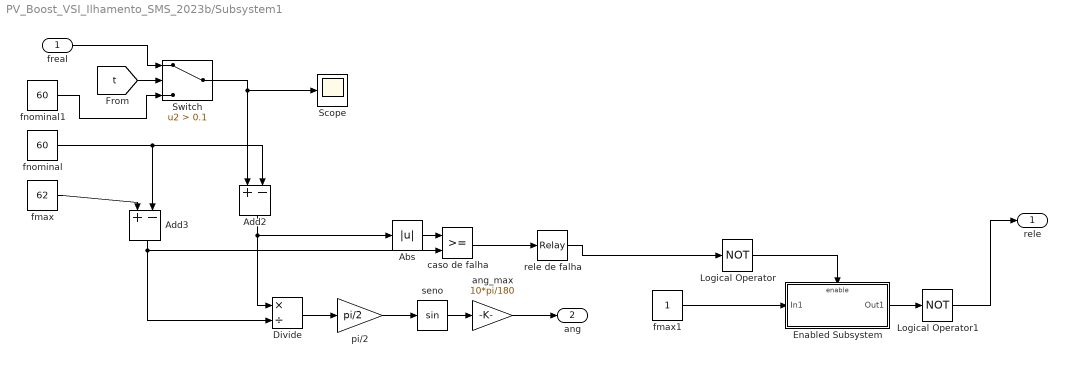
== system PV_Boost_VSI_Ilhamento_SMS_2023b/Subsystem1 ==
  freal : Inport
  Abs : Abs  SaturateOnIntegerOverflow=off
  Add2 : Sum  Inputs=+-
  Add3 : Sum  Inputs=+-
  Divide : Product  Inputs=*/
  Enabled Subsystem : Subsystem  TreatAsAtomicUnit=on
  Logical Operator : Logic  Operator=NOT  AllPortsSameDT=off  OutDataTypeStr=boolean
  Logical Operator1 : Logic  Operator=NOT  AllPortsSameDT=off  OutDataTypeStr=boolean
  Scope : Scope
  Switch : Switch  Criteria=u2 > Threshold  Threshold=0.1  SaturateOnIntegerOverflow=off  InputSameDT=off
  ang_max : Gain  Gain=10*pi/180
  caso de falha : RelationalOperator  OutDataTypeStr=uint(8)  InputSameDT=off
  fmax : Constant  Value=62
  fmax1 : Constant
  fnominal : Constant  Value=60
  fnominal1 : Constant  Value=60
  pi/2 : Gain  Gain=pi/2
  rele de falha : Relay  OnSwitchValue=0.5  OffSwitchValue=0.5  OnOutputValue=0  OffOutputValue=1
  seno : Trigonometry
  rele : Outport
  ang : Outport  Port=2
  wires:
  fnominal/1 -> Add2/2, Add3/2
  fmax/1 -> Add3/1
  Add2/1 -> Divide/1, Abs/1
  Add3/1 -> Divide/2, caso de falha/2
  Divide/1 -> pi/2/1
  pi/2/1 -> seno/1
  Abs/1 -> caso de falha/1
  seno/1 -> ang_max/1
  caso de falha/1 -> rele de falha/1
  ang_max/1 -> ang/1
  rele de falha/1 -> Logical Operator/1
  Enabled Subsystem/1(Out1) -> Logical Operator1/1
  Logical Operator/1 -> Enabled Subsystem/Enable
  fmax1/1 -> Enabled Subsystem/1(In1)
  Logical Operator1/1 -> rele/1
  [t] -> Switch/2
  Switch/1 -> Scope/1, Add2/1
  freal/1 -> Switch/1
  fnominal1/1 -> Switch/3

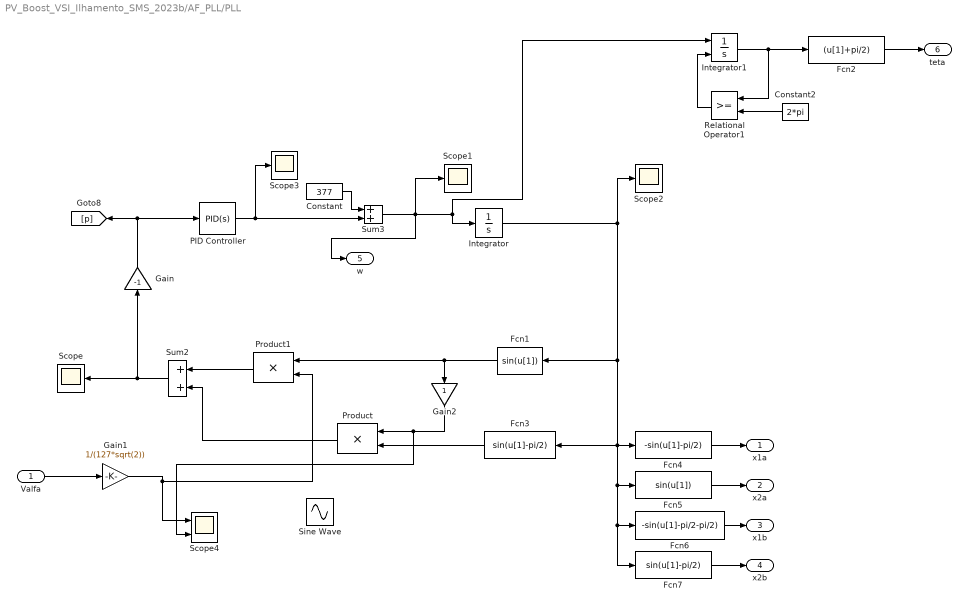
== system PV_Boost_VSI_Ilhamento_SMS_2023b/AF_PLL/PLL ==
  Valfa : Inport
  Constant : Constant  Value=377  SampleTime=-1
  Constant2 : Constant  Value=2*pi
  Fcn1 : Fcn
  Fcn2 : Fcn  Expr=(u[1]+pi/2)
  Fcn3 : Fcn  Expr=sin(u[1]-pi/2)
  Fcn4 : Fcn  Expr=-sin(u[1]-pi/2)
  Fcn5 : Fcn
  Fcn6 : Fcn  Expr=-sin(u[1]-pi/2-pi/2)
  Fcn7 : Fcn  Expr=sin(u[1]-pi/2)
  Gain : Gain  Gain=-1
  Gain1 : Gain  Gain=1/(127*sqrt(2))
  Gain2 : Gain
  Integrator : Integrator
  Integrator1 : Integrator  ExternalReset=rising  InitialCondition=-pi/2
  PID Controller : slpidlib/PID Controller  Controller=PID  Form=Parallel  TimeDomain=Continuous-time  UseExternalTs=off  SampleTime=-1  IntegratorMethod=Forward Euler  FilterMethod=Forward Euler  ControllerParametersSource=internal  P=247.5092  I=10969  UseKiTs=off  D=0  UseExternalDerivativeSource=off  N=100  UseFilter=on  TunerSelectOption=Transfer Function Based (PID Tuner App)  InitialConditionSource=internal  InitialConditionForIntegrator=0  InitialConditionForFilter=0  DifferentiatorICPrevScaledInput=0  ExternalReset=none  TrackingMode=off  Kt=1  LimitOutput=off  SatLimitsSource=internal  UpperSaturationLimit=inf  LowerSaturationLimit=-inf  LinearizeAsGain=on  AntiWindupMode=none  Kb=1  LimitIntegrator=off  UpperIntegratorSaturationLimit=inf  LowerIntegratorSaturationLimit=-inf  POutMin=[]  POutMax=[]  IOutMin=[]  IOutMax=[]  DOutMin=[]  DOutMax=[]  NOutMin=[]  NOutMax=[]  SumOutMin=[]  SumOutMax=[]  SaturationOutMin=[]  SaturationOutMax=[]  PParamMin=[]  PParamMax=[]  IParamMin=[]  IParamMax=[]  DParamMin=[]  DParamMax=[]  NParamMin=[]  NParamMax=[]  KbParamMin=[]  KbParamMax=[]  KtParamMin=[]  KtParamMax=[]  KbOutMin=[]  KbOutMax=[]  KtOutMin=[]  KtOutMax=[]  IntegratorOutMin=[]  IntegratorOutMax=[]  FilterOutMin=[]  FilterOutMax=[]  SumI1OutMin=[]  SumI1OutMax=[]  SumI2OutMin=[]  SumI2OutMax=[]  SumI3OutMin=[]  SumI3OutMax=[]  SumI4OutMin=[]  SumI4OutMax=[]  SumDOutMin=[]  SumDOutMax=[]  DifferentiatorOutMin=[]  DifferentiatorOutMax=[]  FilterDiffOutCoefMin=[]  FilterDiffOutCoefMax=[]  ReciprocalOutMin=[]  ReciprocalOutMax=[]  SumDenOutMin=[]  SumDenOutMax=[]  SumNumOutMin=[]  SumNumOutMax=[]  DivideOutMin=[]  DivideOutMax=[]  UdiffTsProdOutMin=[]  UdiffTsProdOutMax=[]  NTsProdOutMin=[]  NTsProdOutMax=[]  UintegralTsProdOutMin=[]  UintegralTsProdOutMax=[]  UngainTsProdOutMin=[]  UngainTsProdOutMax=[]  ClampingZeroOutDataTypeStr=Inherit: Inherit via back propagation  ClampingZeroOutMin=[]  ClampingZeroOutMax=[]  FilterDenConstantOutDataTypeStr=Inherit: Inherit via back propagation  FilterDenConstantOutMin=[]  FilterDenConstantOutMax=[]  PCopyOutDataTypeStr=Inherit: Inherit via back propagation  PCopyOutMin=[]  PCopyOutMax=[]  NCopyOutDataTypeStr=Inherit: Inherit via back propagation  NCopyOutMin=[]  NCopyOutMax=[]  IntegratorContinuousStateAttributes=''  IntegratorStateMustResolveToSignalObject=off  IntegratorRTWStateStorageClass=Auto  FilterContinuousStateAttributes=''  FilterStateMustResolveToSignalObject=off  FilterRTWStateStorageClass=Auto  ParallelPVariant=InternalParameters  IdealPVariant=Disabled  IVariant=InternalParameters  DVariant=InternalParameters  IntegratorVariant=Continuous  SatVariant=Disabled  AWVariant=Passthrough  PCopyVariant=Disabled  TRVariant=Disabled  FdbkBlocksVariant=Forward  IdealPFdbkVariant=Disabled  SatFdbkVariant=Disabled  DerivativeFilterVariant=ContFilter  NVariant=InternalParameters  NCopyVariant=Disabled  FilterICVariant=InternalICsFilter  IntegratorICVariant=InternalICs  ExternalResetVariant=Disabled  TRSumVariant=Passthrough  SumFdbkVariant=Disabled  SumVariant=Sum_PID  TsampFilterVariant=InternalTs  TsampNgainVariant=Passthrough  TsampIntegralVariant=Disabled_SignalSpec  ExternalSaturationOutDataTypeStr=Inherit: Same as second input  DerivativeSourceVariant=ErrorSignal  PreIntVariant=InternalPreInt
  Product : Product  InputSameDT=on  RndMeth=Zero  SaturateOnIntegerOverflow=on  OutDataTypeStr=Inherit: Same as first input
  Product1 : Product  InputSameDT=on  RndMeth=Zero  SaturateOnIntegerOverflow=on  OutDataTypeStr=Inherit: Same as first input
  Relational Operator1 : RelationalOperator  OutDataTypeStr=boolean  RndMeth=Simplest  InputSameDT=off
  Scope{,1..3} (4 alike) : Scope
  Scope4 : Scope  NumInputPorts=2
  Sine Wave : Sin  Frequency=2*pi*60  SampleTime=0
  Sum2 : Sum  InputSameDT=on  SaturateOnIntegerOverflow=on  OutDataTypeStr=Inherit: Same as first input
  Sum3 : Sum  InputSameDT=on  SaturateOnIntegerOverflow=on  OutDataTypeStr=Inherit: Same as first input
  x1a : Outport
  x2a : Outport  Port=2
  x1b : Outport  Port=3
  x2b : Outport  Port=4
  w : Outport  Port=5
  teta : Outport  Port=6
  wires:
  Product1/1 -> Sum2/1
  Product/1 -> Sum2/2
  Fcn3/1 -> Product/2
  Sum2/1 -> Gain/1, Scope/1
  PID Controller/1 -> Scope3/1, Sum3/2
  Sum3/1 -> w/1, Scope1/1, Integrator1/1, Integrator/1
  Constant/1 -> Sum3/1
  Gain/1 -> PID Controller/1, [p]
  Fcn4/1 -> x1a/1
  Fcn5/1 -> x2a/1
  Fcn6/1 -> x1b/1
  Fcn7/1 -> x2b/1
  Valfa/1 -> Gain1/1
  Fcn1/1 -> Gain2/1, Product1/1
  Integrator/1 -> Fcn3/1, Fcn4/1, Fcn5/1, Fcn6/1, Fcn7/1, Fcn1/1, Scope2/1
  Gain2/1 -> Scope4/2, Product/1
  Gain1/1 -> Product1/2, Scope4/1
  Fcn2/1 -> teta/1
  Integrator1/1 -> Relational Operator1/1, Fcn2/1
  Relational Operator1/1 -> Integrator1/2
  Constant2/1 -> Relational Operator1/2

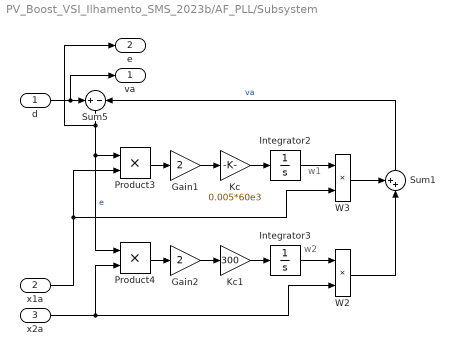
== system PV_Boost_VSI_Ilhamento_SMS_2023b/AF_PLL/Subsystem ==
  note: w2
  note: w1
  d : Inport
  x1a : Inport  Port=2
  x2a : Inport  Port=3
  Gain1 : Gain  Gain=2
  Gain2 : Gain  Gain=2
  Integrator2 : Integrator
  Integrator3 : Integrator
  Kc : Gain  Gain=0.005*60e3
  Kc1 : Gain  Gain=300
  Product3 : Product
  Product4 : Product
  Sum1 : Sum  Inputs=++|
  Sum5 : Sum  Inputs=+-
  W2 : Product
  W3 : Product
  va : Outport
  e : Outport  Port=2
  wires:
  W3/1 -> Sum1/1
  Gain1/1 -> Kc/1
  d/1 -> va/1, Sum5/1
  Integrator2/1 -> W3/1
  Product4/1 -> Gain2/1
  W2/1 -> Sum1/2
  Kc/1 -> Integrator2/1
  Sum1/1 -> Sum5/2  "va"
  Product3/1 -> Gain1/1
  Kc1/1 -> Integrator3/1
  Sum5/1 -> Product4/1, Product3/1, e/1  "e"
  Gain2/1 -> Kc1/1
  Integrator3/1 -> W2/1
  x1a/1 -> Product3/2, W3/2
  x2a/1 -> Product4/2, W2/2

== system PV_Boost_VSI_Ilhamento_SMS_2023b/Subsystem1/Enabled Subsystem ==
  In1 : Inport
  Enable : EnablePort
  Out1 : Outport
  wires:
  In1/1 -> Out1/1

== matlab function PV_Boost_VSI_Ilhamento_SMS_2023b/PV Array/Embedded MATLAB Function ==
  settings: updateMethod=DISCRETE
  data: Vpv input; Ipv output; Psun input; T input
function Ipv = PV_Array(Vpv, Psun, T)
Rs = 0.00305;            %Resistência série da célula
Rp = 18;                %Resistência paralela da célula
Ms = 4;               %Número de módulos em série             
Mp = 1;                %Número de módulos em paralelo
Ns = 60;               %Número de células fotovoltaicas interconectadas (característica do PV)
Voc = 37.5/Ns;         %Tensão de circuito aberto (característica do PV)
Isc = 8.49;            %Corrente de curto-circuito em STC (característica do PV)
a = 3.18e-3;           %Coeficiente de temperatura de Isc(característica do PV)          
n = 1.2;
k = 1.38e-23;
q = 1.60e-19;
EG = 1.1;
Tr = 273 + 25;
T = 273 + T;
Vt = n*k*T/q;
V = Vpv/Ns/Ms;
Iph = (Isc+a*(T-Tr))*Psun/1000;
Irr = (Isc-Voc/Rp)/(exp(q*Voc/n/k/Tr)-1);
Ir = Irr*(T/Tr)^3*exp(q*EG/n/k*(1/Tr-1/T));
I = 0;
for j=1:5;
I = I-(Iph-I-Ir*(exp((V+I*Rs)/Vt)-1)-(V+I*Rs)/Rp)/(-1-Ir*exp((V+I*Rs)/Vt)*Rs/Vt-Rs/Rp);
end
if I<0 I=0;
end
if (I>Isc)
    I=Isc;
end
Ipv = I*Mp;
